simulink model "PVtestsiteeight"  (Simulink 10.1)
settings: Solver=FixedStepDiscrete  StartTime=0.0  StopTime=inf  FixedStep=Ts  RelTol=1e-3
PreLoadFcn:
  | init_DCDCDCAC_new
InitFcn:
  | init_DCDCDCAC_new
undefined symbols (not defined in the file or in its folder): D1, Delta, I, Left, Right, type, V
libraries: powerlib x174, powerlib_meascontrol x3, ssn_lib x2, artemis x1
(part 2 of 3)

== system PVtestsiteeight/SS_Grid/704 - 720 Config 723 ==
  Pi Section Line : powerlib/Elements/Pi Section Line  LConnTagsString=__new0  RConnTagsString=__new0  Frequency=60  Resistance=0.803807  Inductance=0.0011064  Capacitance=1.23355e-07  Length=D  PiSections=1  Measurements=None
      settings: AttributesFormatString=\n  SourceProductBaseCode=PS
  Pi Section Line1 : powerlib/Elements/Pi Section Line  LConnTagsString=__new0  RConnTagsString=__new0  Frequency=60  Resistance=0.80915157  Inductance=0.00104267  Capacitance=1.233552e-07  Length=D  PiSections=1  Measurements=None
      settings: AttributesFormatString=\n  SourceProductBaseCode=PS
  Pi Section Line2 : powerlib/Elements/Pi Section Line  LConnTagsString=__new0  RConnTagsString=__new0  Frequency=60  Resistance=0.8038077  Inductance=0.0011064  Capacitance=1.23355e-07  Length=D  PiSections=1  Measurements=None
      settings: AttributesFormatString=\n  SourceProductBaseCode=PS
  a : PMIOPort  Side=Left
  A : PMIOPort  Port=2  Side=Right
  b : PMIOPort  Port=3  Side=Left
  B : PMIOPort  Port=4  Side=Right
  c : PMIOPort  Port=5  Side=Left
  C : PMIOPort  Port=6  Side=Right
  connections:
  a/RConn1 -- Pi Section Line/LConn1
  A/RConn1 -- Pi Section Line/RConn1
  b/RConn1 -- Pi Section Line1/LConn1
  B/RConn1 -- Pi Section Line1/RConn1
  c/RConn1 -- Pi Section Line2/LConn1
  C/RConn1 -- Pi Section Line2/RConn1

== system PVtestsiteeight/SS_Grid/705 ==
  Three-Phase V-I Measurement : powerlib/Measurements/Three-Phase V-I Measurement  VoltageMeasurement=phase-to-ground  SetLabelV=off  LabelV=Vabc  Vpu=off  VpuLL=off  CurrentMeasurement=yes  SetLabelI=off  LabelI=Iabc  Ipu=off  Pbase=100e6  Vbase=500e3  OutputType=Complex  PhasorSimulation=off  PSBequivalent=0
  Conn1 : PMIOPort  Side=Left
  Conn2 : PMIOPort  Port=2  Side=Left
  Conn3 : PMIOPort  Port=3  Side=Right
  Conn4 : PMIOPort  Port=4  Side=Right
  Conn5 : PMIOPort  Port=5  Side=Left
  Conn6 : PMIOPort  Port=6  Side=Right
  tag scope: I_705=global, V_705=global
  wires:
  Three-Phase V-I Measurement/1 -> [V_705]
  Three-Phase V-I Measurement/2 -> [I_705]
  connections:
  Conn1/RConn1 -- Three-Phase V-I Measurement/LConn1
  Conn2/RConn1 -- Three-Phase V-I Measurement/LConn2
  Conn3/RConn1 -- Three-Phase V-I Measurement/RConn1
  Conn4/RConn1 -- Three-Phase V-I Measurement/RConn2
  Conn5/RConn1 -- Three-Phase V-I Measurement/LConn3
  Conn6/RConn1 -- Three-Phase V-I Measurement/RConn3

== system PVtestsiteeight/SS_Grid/705 - 712 config 724  ==
  Pi Section Line : powerlib/Elements/Pi Section Line  LConnTagsString=__new0  RConnTagsString=__new0  Frequency=60  Resistance=1.3019001  Inductance=0.0012787  Capacitance=9.93038e-08  Length=D  PiSections=1  Measurements=None
      settings: AttributesFormatString=\n  SourceProductBaseCode=PS
  Pi Section Line1 : powerlib/Elements/Pi Section Line  LConnTagsString=__new0  RConnTagsString=__new0  Frequency=60  Resistance=1.309108  Inductance=0.001219369  Capacitance=9.9303e-08  Length=D  PiSections=1  Measurements=None
      settings: AttributesFormatString=\n  SourceProductBaseCode=PS
  Pi Section Line2 : powerlib/Elements/Pi Section Line  LConnTagsString=__new0  RConnTagsString=__new0  Frequency=60  Resistance=1.3019001  Inductance=0.0012787  Capacitance=9.93038e-08  Length=D  PiSections=1  Measurements=None
      settings: AttributesFormatString=\n  SourceProductBaseCode=PS
  a : PMIOPort  Side=Left
  A : PMIOPort  Port=2  Side=Right
  b : PMIOPort  Port=3  Side=Left
  B : PMIOPort  Port=4  Side=Right
  c : PMIOPort  Port=5  Side=Left
  C : PMIOPort  Port=6  Side=Right
  connections:
  a/RConn1 -- Pi Section Line/LConn1
  A/RConn1 -- Pi Section Line/RConn1
  b/RConn1 -- Pi Section Line1/LConn1
  B/RConn1 -- Pi Section Line1/RConn1
  c/RConn1 -- Pi Section Line2/LConn1
  C/RConn1 -- Pi Section Line2/RConn1

== system PVtestsiteeight/SS_Grid/705 - 742 config 724 ==
  Pi Section Line : powerlib/Elements/Pi Section Line  LConnTagsString=__new0  RConnTagsString=__new0  Frequency=60  Resistance=1.3019001  Inductance=0.0012787  Capacitance=9.93038e-08  Length=D  PiSections=1  Measurements=None
      settings: AttributesFormatString=\n  SourceProductBaseCode=PS
  Pi Section Line1 : powerlib/Elements/Pi Section Line  LConnTagsString=__new0  RConnTagsString=__new0  Frequency=60  Resistance=1.309108  Inductance=0.001219369  Capacitance=9.9303e-08  Length=D  PiSections=1  Measurements=None
      settings: AttributesFormatString=\n  SourceProductBaseCode=PS
  Pi Section Line2 : powerlib/Elements/Pi Section Line  LConnTagsString=__new0  RConnTagsString=__new0  Frequency=60  Resistance=1.3019001  Inductance=0.0012787  Capacitance=9.93038e-08  Length=D  PiSections=1  Measurements=None
      settings: AttributesFormatString=\n  SourceProductBaseCode=PS
  a : PMIOPort  Side=Left
  A : PMIOPort  Port=2  Side=Right
  b : PMIOPort  Port=3  Side=Left
  B : PMIOPort  Port=4  Side=Right
  c : PMIOPort  Port=5  Side=Left
  C : PMIOPort  Port=6  Side=Right
  connections:
  C/RConn1 -- Pi Section Line2/RConn1
  c/RConn1 -- Pi Section Line2/LConn1
  B/RConn1 -- Pi Section Line1/RConn1
  b/RConn1 -- Pi Section Line1/LConn1
  A/RConn1 -- Pi Section Line/RConn1
  a/RConn1 -- Pi Section Line/LConn1

== system PVtestsiteeight/SS_Grid/706 ==
  Three-Phase V-I Measurement : powerlib/Measurements/Three-Phase V-I Measurement  VoltageMeasurement=phase-to-ground  SetLabelV=off  LabelV=Vabc  Vpu=off  VpuLL=off  CurrentMeasurement=yes  SetLabelI=off  LabelI=Iabc  Ipu=off  Pbase=100e6  Vbase=500e3  OutputType=Complex  PhasorSimulation=off  PSBequivalent=0
  Conn1 : PMIOPort  Side=Left
  Conn2 : PMIOPort  Port=2  Side=Left
  Conn3 : PMIOPort  Port=3  Side=Right
  Conn4 : PMIOPort  Port=4  Side=Right
  Conn5 : PMIOPort  Port=5  Side=Left
  Conn6 : PMIOPort  Port=6  Side=Right
  tag scope: I_706=global, V_706=global
  wires:
  Three-Phase V-I Measurement/2 -> [I_706]
  Three-Phase V-I Measurement/1 -> [V_706]
  connections:
  Conn6/RConn1 -- Three-Phase V-I Measurement/RConn3
  Conn5/RConn1 -- Three-Phase V-I Measurement/LConn3
  Conn4/RConn1 -- Three-Phase V-I Measurement/RConn2
  Conn3/RConn1 -- Three-Phase V-I Measurement/RConn1
  Conn2/RConn1 -- Three-Phase V-I Measurement/LConn2
  Conn1/RConn1 -- Three-Phase V-I Measurement/LConn1

== system PVtestsiteeight/SS_Grid/706 - 725  config 724 ==
  Pi Section Line : powerlib/Elements/Pi Section Line  LConnTagsString=__new0  RConnTagsString=__new0  Frequency=60  Resistance=1.3019001  Inductance=0.0012787  Capacitance=9.93038e-08  Length=D  PiSections=1  Measurements=None
      settings: AttributesFormatString=\n  SourceProductBaseCode=PS
  Pi Section Line1 : powerlib/Elements/Pi Section Line  LConnTagsString=__new0  RConnTagsString=__new0  Frequency=60  Resistance=1.309108  Inductance=0.001219369  Capacitance=9.9303e-08  Length=D  PiSections=1  Measurements=None
      settings: AttributesFormatString=\n  SourceProductBaseCode=PS
  Pi Section Line2 : powerlib/Elements/Pi Section Line  LConnTagsString=__new0  RConnTagsString=__new0  Frequency=60  Resistance=1.3019001  Inductance=0.0012787  Capacitance=9.93038e-08  Length=D  PiSections=1  Measurements=None
      settings: AttributesFormatString=\n  SourceProductBaseCode=PS
  a : PMIOPort  Side=Left
  A : PMIOPort  Port=2  Side=Right
  b : PMIOPort  Port=3  Side=Left
  B : PMIOPort  Port=4  Side=Right
  c : PMIOPort  Port=5  Side=Left
  C : PMIOPort  Port=6  Side=Right
  connections:
  C/RConn1 -- Pi Section Line2/RConn1
  c/RConn1 -- Pi Section Line2/LConn1
  B/RConn1 -- Pi Section Line1/RConn1
  b/RConn1 -- Pi Section Line1/LConn1
  A/RConn1 -- Pi Section Line/RConn1
  a/RConn1 -- Pi Section Line/LConn1

== system PVtestsiteeight/SS_Grid/707 ==
  Three-Phase V-I Measurement : powerlib/Measurements/Three-Phase V-I Measurement  VoltageMeasurement=phase-to-ground  SetLabelV=off  LabelV=Vabc  Vpu=off  VpuLL=off  CurrentMeasurement=yes  SetLabelI=off  LabelI=Iabc  Ipu=off  Pbase=100e6  Vbase=500e3  OutputType=Complex  PhasorSimulation=off  PSBequivalent=0
  Conn1 : PMIOPort  Side=Left
  Conn2 : PMIOPort  Port=2  Side=Left
  Conn3 : PMIOPort  Port=3  Side=Right
  Conn4 : PMIOPort  Port=4  Side=Right
  Conn5 : PMIOPort  Port=5  Side=Left
  Conn6 : PMIOPort  Port=6  Side=Right
  tag scope: I_707=global, V_707=global
  wires:
  Three-Phase V-I Measurement/1 -> [V_707]
  Three-Phase V-I Measurement/2 -> [I_707]
  connections:
  Conn1/RConn1 -- Three-Phase V-I Measurement/LConn1
  Conn2/RConn1 -- Three-Phase V-I Measurement/LConn2
  Conn3/RConn1 -- Three-Phase V-I Measurement/RConn1
  Conn4/RConn1 -- Three-Phase V-I Measurement/RConn2
  Conn5/RConn1 -- Three-Phase V-I Measurement/LConn3
  Conn6/RConn1 -- Three-Phase V-I Measurement/RConn3

== system PVtestsiteeight/SS_Grid/707 - 722 config 724 ==
  Pi Section Line : powerlib/Elements/Pi Section Line  LConnTagsString=__new0  RConnTagsString=__new0  Frequency=60  Resistance=1.3019001  Inductance=0.0012787  Capacitance=9.93038e-08  Length=D  PiSections=1  Measurements=None
      settings: AttributesFormatString=\n  SourceProductBaseCode=PS
  Pi Section Line1 : powerlib/Elements/Pi Section Line  LConnTagsString=__new0  RConnTagsString=__new0  Frequency=60  Resistance=1.309108  Inductance=0.001219369  Capacitance=9.9303e-08  Length=D  PiSections=1  Measurements=None
      settings: AttributesFormatString=\n  SourceProductBaseCode=PS
  Pi Section Line2 : powerlib/Elements/Pi Section Line  LConnTagsString=__new0  RConnTagsString=__new0  Frequency=60  Resistance=1.3019001  Inductance=0.0012787  Capacitance=9.93038e-08  Length=D  PiSections=1  Measurements=None
      settings: AttributesFormatString=\n  SourceProductBaseCode=PS
  a : PMIOPort  Side=Left
  A : PMIOPort  Port=2  Side=Right
  b : PMIOPort  Port=3  Side=Left
  B : PMIOPort  Port=4  Side=Right
  c : PMIOPort  Port=5  Side=Left
  C : PMIOPort  Port=6  Side=Right
  connections:
  a/RConn1 -- Pi Section Line/LConn1
  A/RConn1 -- Pi Section Line/RConn1
  b/RConn1 -- Pi Section Line1/LConn1
  B/RConn1 -- Pi Section Line1/RConn1
  c/RConn1 -- Pi Section Line2/LConn1
  C/RConn1 -- Pi Section Line2/RConn1

== system PVtestsiteeight/SS_Grid/707 - 724 config 724 ==
  Pi Section Line : powerlib/Elements/Pi Section Line  LConnTagsString=__new0  RConnTagsString=__new0  Frequency=60  Resistance=1.3019001  Inductance=0.0012787  Capacitance=9.93038e-08  Length=D  PiSections=1  Measurements=None
      settings: AttributesFormatString=\n  SourceProductBaseCode=PS
  Pi Section Line1 : powerlib/Elements/Pi Section Line  LConnTagsString=__new0  RConnTagsString=__new0  Frequency=60  Resistance=1.309108  Inductance=0.001219369  Capacitance=9.9303e-08  Length=D  PiSections=1  Measurements=None
      settings: AttributesFormatString=\n  SourceProductBaseCode=PS
  Pi Section Line2 : powerlib/Elements/Pi Section Line  LConnTagsString=__new0  RConnTagsString=__new0  Frequency=60  Resistance=1.3019001  Inductance=0.0012787  Capacitance=9.93038e-08  Length=D  PiSections=1  Measurements=None
      settings: AttributesFormatString=\n  SourceProductBaseCode=PS
  a : PMIOPort  Side=Left
  A : PMIOPort  Port=2  Side=Right
  b : PMIOPort  Port=3  Side=Left
  B : PMIOPort  Port=4  Side=Right
  c : PMIOPort  Port=5  Side=Left
  C : PMIOPort  Port=6  Side=Right
  connections:
  C/RConn1 -- Pi Section Line2/RConn1
  c/RConn1 -- Pi Section Line2/LConn1
  B/RConn1 -- Pi Section Line1/RConn1
  b/RConn1 -- Pi Section Line1/LConn1
  A/RConn1 -- Pi Section Line/RConn1
  a/RConn1 -- Pi Section Line/LConn1

== system PVtestsiteeight/SS_Grid/708 ==
  Three-Phase V-I Measurement : powerlib/Measurements/Three-Phase V-I Measurement  VoltageMeasurement=phase-to-ground  SetLabelV=off  LabelV=Vabc  Vpu=off  VpuLL=off  CurrentMeasurement=yes  SetLabelI=off  LabelI=Iabc  Ipu=off  Pbase=100e6  Vbase=500e3  OutputType=Complex  PhasorSimulation=off  PSBequivalent=0
  Conn1 : PMIOPort  Side=Left
  Conn2 : PMIOPort  Port=2  Side=Left
  Conn3 : PMIOPort  Port=3  Side=Right
  Conn4 : PMIOPort  Port=4  Side=Right
  Conn5 : PMIOPort  Port=5  Side=Left
  Conn6 : PMIOPort  Port=6  Side=Right
  tag scope: I_708=global, V_708=global
  wires:
  Three-Phase V-I Measurement/2 -> [I_708]
  Three-Phase V-I Measurement/1 -> [V_708]
  connections:
  Conn6/RConn1 -- Three-Phase V-I Measurement/RConn3
  Conn5/RConn1 -- Three-Phase V-I Measurement/LConn3
  Conn4/RConn1 -- Three-Phase V-I Measurement/RConn2
  Conn3/RConn1 -- Three-Phase V-I Measurement/RConn1
  Conn2/RConn1 -- Three-Phase V-I Measurement/LConn2
  Conn1/RConn1 -- Three-Phase V-I Measurement/LConn1

== system PVtestsiteeight/SS_Grid/708  - 733 Conf 723 ==
  Pi Section Line : powerlib/Elements/Pi Section Line  LConnTagsString=__new0  RConnTagsString=__new0  Frequency=60  Resistance=0.803807  Inductance=0.0011064  Capacitance=1.23355e-07  Length=D  PiSections=1  Measurements=None
      settings: AttributesFormatString=\n  SourceProductBaseCode=PS
  Pi Section Line1 : powerlib/Elements/Pi Section Line  LConnTagsString=__new0  RConnTagsString=__new0  Frequency=60  Resistance=0.80915157  Inductance=0.00104267  Capacitance=1.233552e-07  Length=D  PiSections=1  Measurements=None
      settings: AttributesFormatString=\n  SourceProductBaseCode=PS
  Pi Section Line2 : powerlib/Elements/Pi Section Line  LConnTagsString=__new0  RConnTagsString=__new0  Frequency=60  Resistance=0.8038077  Inductance=0.0011064  Capacitance=1.23355e-07  Length=D  PiSections=1  Measurements=None
      settings: AttributesFormatString=\n  SourceProductBaseCode=PS
  a : PMIOPort  Side=Left
  A : PMIOPort  Port=2  Side=Right
  b : PMIOPort  Port=3  Side=Left
  B : PMIOPort  Port=4  Side=Right
  c : PMIOPort  Port=5  Side=Left
  C : PMIOPort  Port=6  Side=Right
  connections:
  a/RConn1 -- Pi Section Line/LConn1
  A/RConn1 -- Pi Section Line/RConn1
  b/RConn1 -- Pi Section Line1/LConn1
  B/RConn1 -- Pi Section Line1/RConn1
  c/RConn1 -- Pi Section Line2/LConn1
  C/RConn1 -- Pi Section Line2/RConn1

== system PVtestsiteeight/SS_Grid/708- 732 config 724  ==
  Pi Section Line : powerlib/Elements/Pi Section Line  LConnTagsString=__new0  RConnTagsString=__new0  Frequency=60  Resistance=1.3019001  Inductance=0.0012787  Capacitance=9.93038e-08  Length=D  PiSections=1  Measurements=None
      settings: AttributesFormatString=\n  SourceProductBaseCode=PS
  Pi Section Line1 : powerlib/Elements/Pi Section Line  LConnTagsString=__new0  RConnTagsString=__new0  Frequency=60  Resistance=1.309108  Inductance=0.001219369  Capacitance=9.9303e-08  Length=D  PiSections=1  Measurements=None
      settings: AttributesFormatString=\n  SourceProductBaseCode=PS
  Pi Section Line2 : powerlib/Elements/Pi Section Line  LConnTagsString=__new0  RConnTagsString=__new0  Frequency=60  Resistance=1.3019001  Inductance=0.0012787  Capacitance=9.93038e-08  Length=D  PiSections=1  Measurements=None
      settings: AttributesFormatString=\n  SourceProductBaseCode=PS
  a : PMIOPort  Side=Left
  A : PMIOPort  Port=2  Side=Right
  b : PMIOPort  Port=3  Side=Left
  B : PMIOPort  Port=4  Side=Right
  c : PMIOPort  Port=5  Side=Left
  C : PMIOPort  Port=6  Side=Right
  connections:
  a/RConn1 -- Pi Section Line/LConn1
  A/RConn1 -- Pi Section Line/RConn1
  b/RConn1 -- Pi Section Line1/LConn1
  B/RConn1 -- Pi Section Line1/RConn1
  c/RConn1 -- Pi Section Line2/LConn1
  C/RConn1 -- Pi Section Line2/RConn1

== system PVtestsiteeight/SS_Grid/709 ==
  Three-Phase V-I Measurement : powerlib/Measurements/Three-Phase V-I Measurement  VoltageMeasurement=phase-to-ground  SetLabelV=off  LabelV=Vabc  Vpu=off  VpuLL=off  CurrentMeasurement=yes  SetLabelI=off  LabelI=Iabc  Ipu=off  Pbase=100e6  Vbase=500e3  OutputType=Complex  PhasorSimulation=off  PSBequivalent=0
  Conn1 : PMIOPort  Side=Left
  Conn2 : PMIOPort  Port=2  Side=Left
  Conn3 : PMIOPort  Port=3  Side=Right
  Conn4 : PMIOPort  Port=4  Side=Right
  Conn5 : PMIOPort  Port=5  Side=Left
  Conn6 : PMIOPort  Port=6  Side=Right
  tag scope: I_709=global, V_709=global
  wires:
  Three-Phase V-I Measurement/1 -> [V_709]
  Three-Phase V-I Measurement/2 -> [I_709]
  connections:
  Conn1/RConn1 -- Three-Phase V-I Measurement/LConn1
  Conn2/RConn1 -- Three-Phase V-I Measurement/LConn2
  Conn3/RConn1 -- Three-Phase V-I Measurement/RConn1
  Conn4/RConn1 -- Three-Phase V-I Measurement/RConn2
  Conn5/RConn1 -- Three-Phase V-I Measurement/LConn3
  Conn6/RConn1 -- Three-Phase V-I Measurement/RConn3

== system PVtestsiteeight/SS_Grid/709 - 708 Config 723 ==
  Pi Section Line : powerlib/Elements/Pi Section Line  LConnTagsString=__new0  RConnTagsString=__new0  Frequency=60  Resistance=0.803807  Inductance=0.0011064  Capacitance=1.23355e-07  Length=D  PiSections=1  Measurements=None
      settings: AttributesFormatString=\n  SourceProductBaseCode=PS
  Pi Section Line1 : powerlib/Elements/Pi Section Line  LConnTagsString=__new0  RConnTagsString=__new0  Frequency=60  Resistance=0.80915157  Inductance=0.00104267  Capacitance=1.233552e-07  Length=D  PiSections=1  Measurements=None
      settings: AttributesFormatString=\n  SourceProductBaseCode=PS
  Pi Section Line2 : powerlib/Elements/Pi Section Line  LConnTagsString=__new0  RConnTagsString=__new0  Frequency=60  Resistance=0.8038077  Inductance=0.0011064  Capacitance=1.23355e-07  Length=D  PiSections=1  Measurements=None
      settings: AttributesFormatString=\n  SourceProductBaseCode=PS
  a : PMIOPort  Side=Left
  A : PMIOPort  Port=2  Side=Right
  b : PMIOPort  Port=3  Side=Left
  B : PMIOPort  Port=4  Side=Right
  c : PMIOPort  Port=5  Side=Left
  C : PMIOPort  Port=6  Side=Right
  connections:
  C/RConn1 -- Pi Section Line2/RConn1
  c/RConn1 -- Pi Section Line2/LConn1
  B/RConn1 -- Pi Section Line1/RConn1
  b/RConn1 -- Pi Section Line1/LConn1
  A/RConn1 -- Pi Section Line/RConn1
  a/RConn1 -- Pi Section Line/LConn1

== system PVtestsiteeight/SS_Grid/709 - 731 Config 723 ==
  Pi Section Line : powerlib/Elements/Pi Section Line  LConnTagsString=__new0  RConnTagsString=__new0  Frequency=60  Resistance=0.803807  Inductance=0.0011064  Capacitance=1.23355e-07  Length=D  PiSections=1  Measurements=None
      settings: AttributesFormatString=\n  SourceProductBaseCode=PS
  Pi Section Line1 : powerlib/Elements/Pi Section Line  LConnTagsString=__new0  RConnTagsString=__new0  Frequency=60  Resistance=0.80915157  Inductance=0.00104267  Capacitance=1.233552e-07  Length=D  PiSections=1  Measurements=None
      settings: AttributesFormatString=\n  SourceProductBaseCode=PS
  Pi Section Line2 : powerlib/Elements/Pi Section Line  LConnTagsString=__new0  RConnTagsString=__new0  Frequency=60  Resistance=0.8038077  Inductance=0.0011064  Capacitance=1.23355e-07  Length=D  PiSections=1  Measurements=None
      settings: AttributesFormatString=\n  SourceProductBaseCode=PS
  a : PMIOPort  Side=Left
  A : PMIOPort  Port=2  Side=Right
  b : PMIOPort  Port=3  Side=Left
  B : PMIOPort  Port=4  Side=Right
  c : PMIOPort  Port=5  Side=Left
  C : PMIOPort  Port=6  Side=Right
  connections:
  a/RConn1 -- Pi Section Line/LConn1
  A/RConn1 -- Pi Section Line/RConn1
  b/RConn1 -- Pi Section Line1/LConn1
  B/RConn1 -- Pi Section Line1/RConn1
  c/RConn1 -- Pi Section Line2/LConn1
  C/RConn1 -- Pi Section Line2/RConn1

== system PVtestsiteeight/SS_Grid/710 ==
  Three-Phase V-I Measurement : powerlib/Measurements/Three-Phase V-I Measurement  VoltageMeasurement=phase-to-ground  SetLabelV=off  LabelV=Vabc  Vpu=off  VpuLL=off  CurrentMeasurement=yes  SetLabelI=off  LabelI=Iabc  Ipu=off  Pbase=100e6  Vbase=500e3  OutputType=Complex  PhasorSimulation=off  PSBequivalent=0
  Conn1 : PMIOPort  Side=Left
  Conn2 : PMIOPort  Port=2  Side=Left
  Conn3 : PMIOPort  Port=3  Side=Right
  Conn4 : PMIOPort  Port=4  Side=Right
  Conn5 : PMIOPort  Port=5  Side=Left
  Conn6 : PMIOPort  Port=6  Side=Right
  tag scope: I_710=global, V_710=global
  wires:
  Three-Phase V-I Measurement/2 -> [I_710]
  Three-Phase V-I Measurement/1 -> [V_710]
  connections:
  Conn6/RConn1 -- Three-Phase V-I Measurement/RConn3
  Conn5/RConn1 -- Three-Phase V-I Measurement/LConn3
  Conn4/RConn1 -- Three-Phase V-I Measurement/RConn2
  Conn3/RConn1 -- Three-Phase V-I Measurement/RConn1
  Conn2/RConn1 -- Three-Phase V-I Measurement/LConn2
  Conn1/RConn1 -- Three-Phase V-I Measurement/LConn1

== system PVtestsiteeight/SS_Grid/710 - 735 config 724  ==
  Pi Section Line : powerlib/Elements/Pi Section Line  LConnTagsString=__new0  RConnTagsString=__new0  Frequency=60  Resistance=1.3019001  Inductance=0.0012787  Capacitance=9.93038e-08  Length=D  PiSections=1  Measurements=None
      settings: AttributesFormatString=\n  SourceProductBaseCode=PS
  Pi Section Line1 : powerlib/Elements/Pi Section Line  LConnTagsString=__new0  RConnTagsString=__new0  Frequency=60  Resistance=1.309108  Inductance=0.001219369  Capacitance=9.9303e-08  Length=D  PiSections=1  Measurements=None
      settings: AttributesFormatString=\n  SourceProductBaseCode=PS
  Pi Section Line2 : powerlib/Elements/Pi Section Line  LConnTagsString=__new0  RConnTagsString=__new0  Frequency=60  Resistance=1.3019001  Inductance=0.0012787  Capacitance=9.93038e-08  Length=D  PiSections=1  Measurements=None
      settings: AttributesFormatString=\n  SourceProductBaseCode=PS
  a : PMIOPort  Side=Left
  A : PMIOPort  Port=2  Side=Right
  b : PMIOPort  Port=3  Side=Left
  B : PMIOPort  Port=4  Side=Right
  c : PMIOPort  Port=5  Side=Left
  C : PMIOPort  Port=6  Side=Right
  connections:
  C/RConn1 -- Pi Section Line2/RConn1
  c/RConn1 -- Pi Section Line2/LConn1
  B/RConn1 -- Pi Section Line1/RConn1
  b/RConn1 -- Pi Section Line1/LConn1
  A/RConn1 -- Pi Section Line/RConn1
  a/RConn1 -- Pi Section Line/LConn1

== system PVtestsiteeight/SS_Grid/710 - 736 config 724  ==
  Pi Section Line : powerlib/Elements/Pi Section Line  LConnTagsString=__new0  RConnTagsString=__new0  Frequency=60  Resistance=1.3019001  Inductance=0.0012787  Capacitance=9.93038e-08  Length=D  PiSections=1  Measurements=None
      settings: AttributesFormatString=\n  SourceProductBaseCode=PS
  Pi Section Line1 : powerlib/Elements/Pi Section Line  LConnTagsString=__new0  RConnTagsString=__new0  Frequency=60  Resistance=1.309108  Inductance=0.001219369  Capacitance=9.9303e-08  Length=D  PiSections=1  Measurements=None
      settings: AttributesFormatString=\n  SourceProductBaseCode=PS
  Pi Section Line2 : powerlib/Elements/Pi Section Line  LConnTagsString=__new0  RConnTagsString=__new0  Frequency=60  Resistance=1.3019001  Inductance=0.0012787  Capacitance=9.93038e-08  Length=D  PiSections=1  Measurements=None
      settings: AttributesFormatString=\n  SourceProductBaseCode=PS
  a : PMIOPort  Side=Left
  A : PMIOPort  Port=2  Side=Right
  b : PMIOPort  Port=3  Side=Left
  B : PMIOPort  Port=4  Side=Right
  c : PMIOPort  Port=5  Side=Left
  C : PMIOPort  Port=6  Side=Right
  connections:
  C/RConn1 -- Pi Section Line2/RConn1
  c/RConn1 -- Pi Section Line2/LConn1
  B/RConn1 -- Pi Section Line1/RConn1
  b/RConn1 -- Pi Section Line1/LConn1
  A/RConn1 -- Pi Section Line/RConn1
  a/RConn1 -- Pi Section Line/LConn1

== system PVtestsiteeight/SS_Grid/711 ==
  Three-Phase V-I Measurement : powerlib/Measurements/Three-Phase V-I Measurement  VoltageMeasurement=phase-to-ground  SetLabelV=off  LabelV=Vabc  Vpu=off  VpuLL=off  CurrentMeasurement=yes  SetLabelI=off  LabelI=Iabc  Ipu=off  Pbase=100e6  Vbase=500e3  OutputType=Complex  PhasorSimulation=off  PSBequivalent=0
  Conn1 : PMIOPort  Side=Left
  Conn2 : PMIOPort  Port=2  Side=Left
  Conn3 : PMIOPort  Port=3  Side=Right
  Conn4 : PMIOPort  Port=4  Side=Right
  Conn5 : PMIOPort  Port=5  Side=Left
  Conn6 : PMIOPort  Port=6  Side=Right
  tag scope: I_711=global, V_711=global
  wires:
  Three-Phase V-I Measurement/1 -> [V_711]
  Three-Phase V-I Measurement/2 -> [I_711]
  connections:
  Conn1/RConn1 -- Three-Phase V-I Measurement/LConn1
  Conn2/RConn1 -- Three-Phase V-I Measurement/LConn2
  Conn3/RConn1 -- Three-Phase V-I Measurement/RConn1
  Conn4/RConn1 -- Three-Phase V-I Measurement/RConn2
  Conn5/RConn1 -- Three-Phase V-I Measurement/LConn3
  Conn6/RConn1 -- Three-Phase V-I Measurement/RConn3

== system PVtestsiteeight/SS_Grid/711 - 740 config 724  ==
  Pi Section Line : powerlib/Elements/Pi Section Line  LConnTagsString=__new0  RConnTagsString=__new0  Frequency=60  Resistance=1.3019001  Inductance=0.0012787  Capacitance=9.93038e-08  Length=D  PiSections=1  Measurements=None
      settings: AttributesFormatString=\n  SourceProductBaseCode=PS
  Pi Section Line1 : powerlib/Elements/Pi Section Line  LConnTagsString=__new0  RConnTagsString=__new0  Frequency=60  Resistance=1.309108  Inductance=0.001219369  Capacitance=9.9303e-08  Length=D  PiSections=1  Measurements=None
      settings: AttributesFormatString=\n  SourceProductBaseCode=PS
  Pi Section Line2 : powerlib/Elements/Pi Section Line  LConnTagsString=__new0  RConnTagsString=__new0  Frequency=60  Resistance=1.3019001  Inductance=0.0012787  Capacitance=9.93038e-08  Length=D  PiSections=1  Measurements=None
      settings: AttributesFormatString=\n  SourceProductBaseCode=PS
  a : PMIOPort  Side=Left
  A : PMIOPort  Port=2  Side=Right
  b : PMIOPort  Port=3  Side=Left
  B : PMIOPort  Port=4  Side=Right
  c : PMIOPort  Port=5  Side=Left
  C : PMIOPort  Port=6  Side=Right
  connections:
  a/RConn1 -- Pi Section Line/LConn1
  A/RConn1 -- Pi Section Line/RConn1
  b/RConn1 -- Pi Section Line1/LConn1
  B/RConn1 -- Pi Section Line1/RConn1
  c/RConn1 -- Pi Section Line2/LConn1
  C/RConn1 -- Pi Section Line2/RConn1

== system PVtestsiteeight/SS_Grid/711 - 741 Conf 723  ==
  Pi Section Line : powerlib/Elements/Pi Section Line  LConnTagsString=__new0  RConnTagsString=__new0  Frequency=60  Resistance=0.803807  Inductance=0.0011064  Capacitance=1.23355e-07  Length=D  PiSections=1  Measurements=None
      settings: AttributesFormatString=\n  SourceProductBaseCode=PS
  Pi Section Line1 : powerlib/Elements/Pi Section Line  LConnTagsString=__new0  RConnTagsString=__new0  Frequency=60  Resistance=0.80915157  Inductance=0.00104267  Capacitance=1.233552e-07  Length=D  PiSections=1  Measurements=None
      settings: AttributesFormatString=\n  SourceProductBaseCode=PS
  Pi Section Line2 : powerlib/Elements/Pi Section Line  LConnTagsString=__new0  RConnTagsString=__new0  Frequency=60  Resistance=0.8038077  Inductance=0.0011064  Capacitance=1.23355e-07  Length=D  PiSections=1  Measurements=None
      settings: AttributesFormatString=\n  SourceProductBaseCode=PS
  a : PMIOPort  Side=Left
  A : PMIOPort  Port=2  Side=Right
  b : PMIOPort  Port=3  Side=Left
  B : PMIOPort  Port=4  Side=Right
  c : PMIOPort  Port=5  Side=Left
  C : PMIOPort  Port=6  Side=Right
  connections:
  C/RConn1 -- Pi Section Line2/RConn1
  c/RConn1 -- Pi Section Line2/LConn1
  B/RConn1 -- Pi Section Line1/RConn1
  b/RConn1 -- Pi Section Line1/LConn1
  A/RConn1 -- Pi Section Line/RConn1
  a/RConn1 -- Pi Section Line/LConn1

== system PVtestsiteeight/SS_Grid/712 ==
  Three-Phase V-I Measurement : powerlib/Measurements/Three-Phase V-I Measurement  VoltageMeasurement=phase-to-ground  SetLabelV=off  LabelV=Vabc  Vpu=off  VpuLL=off  CurrentMeasurement=yes  SetLabelI=off  LabelI=Iabc  Ipu=off  Pbase=100e6  Vbase=500e3  OutputType=Complex  PhasorSimulation=off  PSBequivalent=0
  Conn1 : PMIOPort  Side=Left
  Conn2 : PMIOPort  Port=2  Side=Left
  Conn3 : PMIOPort  Port=3  Side=Right
  Conn4 : PMIOPort  Port=4  Side=Right
  Conn5 : PMIOPort  Port=5  Side=Left
  Conn6 : PMIOPort  Port=6  Side=Right
  tag scope: I_712=global, V_712=global
  wires:
  Three-Phase V-I Measurement/1 -> [V_712]
  Three-Phase V-I Measurement/2 -> [I_712]
  connections:
  Conn1/RConn1 -- Three-Phase V-I Measurement/LConn1
  Conn2/RConn1 -- Three-Phase V-I Measurement/LConn2
  Conn3/RConn1 -- Three-Phase V-I Measurement/RConn1
  Conn4/RConn1 -- Three-Phase V-I Measurement/RConn2
  Conn5/RConn1 -- Three-Phase V-I Measurement/LConn3
  Conn6/RConn1 -- Three-Phase V-I Measurement/RConn3

== system PVtestsiteeight/SS_Grid/713 ==
  Three-Phase V-I Measurement : powerlib/Measurements/Three-Phase V-I Measurement  VoltageMeasurement=phase-to-ground  SetLabelV=off  LabelV=Vabc  Vpu=off  VpuLL=off  CurrentMeasurement=yes  SetLabelI=off  LabelI=Iabc  Ipu=off  Pbase=100e6  Vbase=500e3  OutputType=Complex  PhasorSimulation=off  PSBequivalent=0
  Conn1 : PMIOPort  Side=Left
  Conn2 : PMIOPort  Port=2  Side=Left
  Conn3 : PMIOPort  Port=3  Side=Right
  Conn4 : PMIOPort  Port=4  Side=Right
  Conn5 : PMIOPort  Port=5  Side=Left
  Conn6 : PMIOPort  Port=6  Side=Right
  tag scope: I_713=global, V_713=global
  wires:
  Three-Phase V-I Measurement/1 -> [V_713]
  Three-Phase V-I Measurement/2 -> [I_713]
  connections:
  Conn1/RConn1 -- Three-Phase V-I Measurement/LConn1
  Conn2/RConn1 -- Three-Phase V-I Measurement/LConn2
  Conn3/RConn1 -- Three-Phase V-I Measurement/RConn1
  Conn4/RConn1 -- Three-Phase V-I Measurement/RConn2
  Conn5/RConn1 -- Three-Phase V-I Measurement/LConn3
  Conn6/RConn1 -- Three-Phase V-I Measurement/RConn3

== system PVtestsiteeight/SS_Grid/713 - 704 Config 723 ==
  Pi Section Line : powerlib/Elements/Pi Section Line  LConnTagsString=__new0  RConnTagsString=__new0  Frequency=60  Resistance=0.803807  Inductance=0.0011064  Capacitance=1.23355e-07  Length=D  PiSections=1  Measurements=None
      settings: AttributesFormatString=\n  SourceProductBaseCode=PS
  Pi Section Line1 : powerlib/Elements/Pi Section Line  LConnTagsString=__new0  RConnTagsString=__new0  Frequency=60  Resistance=0.80915157  Inductance=0.00104267  Capacitance=1.233552e-07  Length=D  PiSections=1  Measurements=None
      settings: AttributesFormatString=\n  SourceProductBaseCode=PS
  Pi Section Line2 : powerlib/Elements/Pi Section Line  LConnTagsString=__new0  RConnTagsString=__new0  Frequency=60  Resistance=0.8038077  Inductance=0.0011064  Capacitance=1.23355e-07  Length=D  PiSections=1  Measurements=None
      settings: AttributesFormatString=\n  SourceProductBaseCode=PS
  a : PMIOPort  Side=Left
  A : PMIOPort  Port=2  Side=Right
  b : PMIOPort  Port=3  Side=Left
  B : PMIOPort  Port=4  Side=Right
  c : PMIOPort  Port=5  Side=Left
  C : PMIOPort  Port=6  Side=Right
  connections:
  C/RConn1 -- Pi Section Line2/RConn1
  c/RConn1 -- Pi Section Line2/LConn1
  B/RConn1 -- Pi Section Line1/RConn1
  b/RConn1 -- Pi Section Line1/LConn1
  A/RConn1 -- Pi Section Line/RConn1
  a/RConn1 -- Pi Section Line/LConn1

== system PVtestsiteeight/SS_Grid/714 ==
  Three-Phase V-I Measurement : powerlib/Measurements/Three-Phase V-I Measurement  VoltageMeasurement=phase-to-ground  SetLabelV=off  LabelV=Vabc  Vpu=off  VpuLL=off  CurrentMeasurement=yes  SetLabelI=off  LabelI=Iabc  Ipu=off  Pbase=100e6  Vbase=500e3  OutputType=Complex  PhasorSimulation=off  PSBequivalent=0
  Conn1 : PMIOPort  Side=Left
  Conn2 : PMIOPort  Port=2  Side=Left
  Conn3 : PMIOPort  Port=3  Side=Right
  Conn4 : PMIOPort  Port=4  Side=Right
  Conn5 : PMIOPort  Port=5  Side=Left
  Conn6 : PMIOPort  Port=6  Side=Right
  tag scope: I_714=global, V_714=global
  wires:
  Three-Phase V-I Measurement/1 -> [V_714]
  Three-Phase V-I Measurement/2 -> [I_714]
  connections:
  Conn1/RConn1 -- Three-Phase V-I Measurement/LConn1
  Conn2/RConn1 -- Three-Phase V-I Measurement/LConn2
  Conn3/RConn1 -- Three-Phase V-I Measurement/RConn1
  Conn4/RConn1 -- Three-Phase V-I Measurement/RConn2
  Conn5/RConn1 -- Three-Phase V-I Measurement/LConn3
  Conn6/RConn1 -- Three-Phase V-I Measurement/RConn3

== system PVtestsiteeight/SS_Grid/714 - 718  config 724 ==
  Pi Section Line : powerlib/Elements/Pi Section Line  LConnTagsString=__new0  RConnTagsString=__new0  Frequency=60  Resistance=1.3019001  Inductance=0.0012787  Capacitance=9.93038e-08  Length=D  PiSections=1  Measurements=None
      settings: AttributesFormatString=\n  SourceProductBaseCode=PS
  Pi Section Line1 : powerlib/Elements/Pi Section Line  LConnTagsString=__new0  RConnTagsString=__new0  Frequency=60  Resistance=1.309108  Inductance=0.001219369  Capacitance=9.9303e-08  Length=D  PiSections=1  Measurements=None
      settings: AttributesFormatString=\n  SourceProductBaseCode=PS
  Pi Section Line2 : powerlib/Elements/Pi Section Line  LConnTagsString=__new0  RConnTagsString=__new0  Frequency=60  Resistance=1.3019001  Inductance=0.0012787  Capacitance=9.93038e-08  Length=D  PiSections=1  Measurements=None
      settings: AttributesFormatString=\n  SourceProductBaseCode=PS
  a : PMIOPort  Side=Left
  A : PMIOPort  Port=2  Side=Right
  b : PMIOPort  Port=3  Side=Left
  B : PMIOPort  Port=4  Side=Right
  c : PMIOPort  Port=5  Side=Left
  C : PMIOPort  Port=6  Side=Right
  connections:
  a/RConn1 -- Pi Section Line/LConn1
  A/RConn1 -- Pi Section Line/RConn1
  b/RConn1 -- Pi Section Line1/LConn1
  B/RConn1 -- Pi Section Line1/RConn1
  c/RConn1 -- Pi Section Line2/LConn1
  C/RConn1 -- Pi Section Line2/RConn1

== system PVtestsiteeight/SS_Grid/718 ==
  Three-Phase V-I Measurement : powerlib/Measurements/Three-Phase V-I Measurement  VoltageMeasurement=phase-to-ground  SetLabelV=off  LabelV=Vabc  Vpu=off  VpuLL=off  CurrentMeasurement=yes  SetLabelI=off  LabelI=Iabc  Ipu=off  Pbase=100e6  Vbase=500e3  OutputType=Complex  PhasorSimulation=off  PSBequivalent=0
  Conn1 : PMIOPort  Side=Left
  Conn2 : PMIOPort  Port=2  Side=Left
  Conn3 : PMIOPort  Port=3  Side=Right
  Conn4 : PMIOPort  Port=4  Side=Right
  Conn5 : PMIOPort  Port=5  Side=Left
  Conn6 : PMIOPort  Port=6  Side=Right
  tag scope: I_718=global, V_718=global
  wires:
  Three-Phase V-I Measurement/2 -> [I_718]
  Three-Phase V-I Measurement/1 -> [V_718]
  connections:
  Conn6/RConn1 -- Three-Phase V-I Measurement/RConn3
  Conn5/RConn1 -- Three-Phase V-I Measurement/LConn3
  Conn4/RConn1 -- Three-Phase V-I Measurement/RConn2
  Conn3/RConn1 -- Three-Phase V-I Measurement/RConn1
  Conn2/RConn1 -- Three-Phase V-I Measurement/LConn2
  Conn1/RConn1 -- Three-Phase V-I Measurement/LConn1

== system PVtestsiteeight/SS_Grid/720 ==
  Three-Phase V-I Measurement : powerlib/Measurements/Three-Phase V-I Measurement  VoltageMeasurement=phase-to-ground  SetLabelV=off  LabelV=Vabc  Vpu=off  VpuLL=off  CurrentMeasurement=yes  SetLabelI=off  LabelI=Iabc  Ipu=off  Pbase=100e6  Vbase=500e3  OutputType=Complex  PhasorSimulation=off  PSBequivalent=0
  Conn1 : PMIOPort  Side=Left
  Conn2 : PMIOPort  Port=2  Side=Left
  Conn3 : PMIOPort  Port=3  Side=Right
  Conn4 : PMIOPort  Port=4  Side=Right
  Conn5 : PMIOPort  Port=5  Side=Left
  Conn6 : PMIOPort  Port=6  Side=Right
  tag scope: I_720=global, V_720=global
  wires:
  Three-Phase V-I Measurement/1 -> [V_720]
  Three-Phase V-I Measurement/2 -> [I_720]
  connections:
  Conn1/RConn1 -- Three-Phase V-I Measurement/LConn1
  Conn2/RConn1 -- Three-Phase V-I Measurement/LConn2
  Conn3/RConn1 -- Three-Phase V-I Measurement/RConn1
  Conn4/RConn1 -- Three-Phase V-I Measurement/RConn2
  Conn5/RConn1 -- Three-Phase V-I Measurement/LConn3
  Conn6/RConn1 -- Three-Phase V-I Measurement/RConn3

== system PVtestsiteeight/SS_Grid/720  - 706 Config 723 ==
  Pi Section Line : powerlib/Elements/Pi Section Line  LConnTagsString=__new0  RConnTagsString=__new0  Frequency=60  Resistance=0.803807  Inductance=0.0011064  Capacitance=1.23355e-07  Length=D  PiSections=1  Measurements=None
      settings: AttributesFormatString=\n  SourceProductBaseCode=PS
  Pi Section Line1 : powerlib/Elements/Pi Section Line  LConnTagsString=__new0  RConnTagsString=__new0  Frequency=60  Resistance=0.80915157  Inductance=0.00104267  Capacitance=1.233552e-07  Length=D  PiSections=1  Measurements=None
      settings: AttributesFormatString=\n  SourceProductBaseCode=PS
  Pi Section Line2 : powerlib/Elements/Pi Section Line  LConnTagsString=__new0  RConnTagsString=__new0  Frequency=60  Resistance=0.8038077  Inductance=0.0011064  Capacitance=1.23355e-07  Length=D  PiSections=1  Measurements=None
      settings: AttributesFormatString=\n  SourceProductBaseCode=PS
  a : PMIOPort  Side=Left
  A : PMIOPort  Port=2  Side=Right
  b : PMIOPort  Port=3  Side=Left
  B : PMIOPort  Port=4  Side=Right
  c : PMIOPort  Port=5  Side=Left
  C : PMIOPort  Port=6  Side=Right
  connections:
  C/RConn1 -- Pi Section Line2/RConn1
  c/RConn1 -- Pi Section Line2/LConn1
  B/RConn1 -- Pi Section Line1/RConn1
  b/RConn1 -- Pi Section Line1/LConn1
  A/RConn1 -- Pi Section Line/RConn1
  a/RConn1 -- Pi Section Line/LConn1

== system PVtestsiteeight/SS_Grid/720 - 707  config 724 ==
  Pi Section Line : powerlib/Elements/Pi Section Line  LConnTagsString=__new0  RConnTagsString=__new0  Frequency=60  Resistance=1.3019001  Inductance=0.0012787  Capacitance=9.93038e-08  Length=D  PiSections=1  Measurements=None
      settings: AttributesFormatString=\n  SourceProductBaseCode=PS
  Pi Section Line1 : powerlib/Elements/Pi Section Line  LConnTagsString=__new0  RConnTagsString=__new0  Frequency=60  Resistance=1.309108  Inductance=0.001219369  Capacitance=9.9303e-08  Length=D  PiSections=1  Measurements=None
      settings: AttributesFormatString=\n  SourceProductBaseCode=PS
  Pi Section Line2 : powerlib/Elements/Pi Section Line  LConnTagsString=__new0  RConnTagsString=__new0  Frequency=60  Resistance=1.3019001  Inductance=0.0012787  Capacitance=9.93038e-08  Length=D  PiSections=1  Measurements=None
      settings: AttributesFormatString=\n  SourceProductBaseCode=PS
  a : PMIOPort  Side=Left
  A : PMIOPort  Port=2  Side=Right
  b : PMIOPort  Port=3  Side=Left
  B : PMIOPort  Port=4  Side=Right
  c : PMIOPort  Port=5  Side=Left
  C : PMIOPort  Port=6  Side=Right
  connections:
  a/RConn1 -- Pi Section Line/LConn1
  A/RConn1 -- Pi Section Line/RConn1
  b/RConn1 -- Pi Section Line1/LConn1
  B/RConn1 -- Pi Section Line1/RConn1
  c/RConn1 -- Pi Section Line2/LConn1
  C/RConn1 -- Pi Section Line2/RConn1

== system PVtestsiteeight/SS_Grid/722 ==
  Three-Phase V-I Measurement : powerlib/Measurements/Three-Phase V-I Measurement  VoltageMeasurement=phase-to-ground  SetLabelV=off  LabelV=Vabc  Vpu=off  VpuLL=off  CurrentMeasurement=yes  SetLabelI=off  LabelI=Iabc  Ipu=off  Pbase=100e6  Vbase=500e3  OutputType=Complex  PhasorSimulation=off  PSBequivalent=0
  Conn1 : PMIOPort  Side=Left
  Conn2 : PMIOPort  Port=2  Side=Left
  Conn3 : PMIOPort  Port=3  Side=Right
  Conn4 : PMIOPort  Port=4  Side=Right
  Conn5 : PMIOPort  Port=5  Side=Left
  Conn6 : PMIOPort  Port=6  Side=Right
  tag scope: I_722=global, V_722=global
  wires:
  Three-Phase V-I Measurement/2 -> [I_722]
  Three-Phase V-I Measurement/1 -> [V_722]
  connections:
  Conn6/RConn1 -- Three-Phase V-I Measurement/RConn3
  Conn5/RConn1 -- Three-Phase V-I Measurement/LConn3
  Conn4/RConn1 -- Three-Phase V-I Measurement/RConn2
  Conn3/RConn1 -- Three-Phase V-I Measurement/RConn1
  Conn2/RConn1 -- Three-Phase V-I Measurement/LConn2
  Conn1/RConn1 -- Three-Phase V-I Measurement/LConn1

== system PVtestsiteeight/SS_Grid/724 ==
  Three-Phase V-I Measurement : powerlib/Measurements/Three-Phase V-I Measurement  VoltageMeasurement=phase-to-ground  SetLabelV=off  LabelV=Vabc  Vpu=off  VpuLL=off  CurrentMeasurement=yes  SetLabelI=off  LabelI=Iabc  Ipu=off  Pbase=100e6  Vbase=500e3  OutputType=Complex  PhasorSimulation=off  PSBequivalent=0
  Conn1 : PMIOPort  Side=Left
  Conn2 : PMIOPort  Port=2  Side=Left
  Conn3 : PMIOPort  Port=3  Side=Right
  Conn4 : PMIOPort  Port=4  Side=Right
  Conn5 : PMIOPort  Port=5  Side=Left
  Conn6 : PMIOPort  Port=6  Side=Right
  tag scope: I_724=global, V_724=global
  wires:
  Three-Phase V-I Measurement/2 -> [I_724]
  Three-Phase V-I Measurement/1 -> [V_724]
  connections:
  Conn6/RConn1 -- Three-Phase V-I Measurement/RConn3
  Conn5/RConn1 -- Three-Phase V-I Measurement/LConn3
  Conn4/RConn1 -- Three-Phase V-I Measurement/RConn2
  Conn3/RConn1 -- Three-Phase V-I Measurement/RConn1
  Conn2/RConn1 -- Three-Phase V-I Measurement/LConn2
  Conn1/RConn1 -- Three-Phase V-I Measurement/LConn1

== system PVtestsiteeight/SS_Grid/725 ==
  Three-Phase V-I Measurement : powerlib/Measurements/Three-Phase V-I Measurement  VoltageMeasurement=phase-to-ground  SetLabelV=off  LabelV=Vabc  Vpu=off  VpuLL=off  CurrentMeasurement=yes  SetLabelI=off  LabelI=Iabc  Ipu=off  Pbase=100e6  Vbase=500e3  OutputType=Complex  PhasorSimulation=off  PSBequivalent=0
  Conn1 : PMIOPort  Side=Left
  Conn2 : PMIOPort  Port=2  Side=Left
  Conn3 : PMIOPort  Port=3  Side=Right
  Conn4 : PMIOPort  Port=4  Side=Right
  Conn5 : PMIOPort  Port=5  Side=Left
  Conn6 : PMIOPort  Port=6  Side=Right
  tag scope: I_725=global, V_725=global
  wires:
  Three-Phase V-I Measurement/1 -> [V_725]
  Three-Phase V-I Measurement/2 -> [I_725]
  connections:
  Conn1/RConn1 -- Three-Phase V-I Measurement/LConn1
  Conn2/RConn1 -- Three-Phase V-I Measurement/LConn2
  Conn3/RConn1 -- Three-Phase V-I Measurement/RConn1
  Conn4/RConn1 -- Three-Phase V-I Measurement/RConn2
  Conn5/RConn1 -- Three-Phase V-I Measurement/LConn3
  Conn6/RConn1 -- Three-Phase V-I Measurement/RConn3

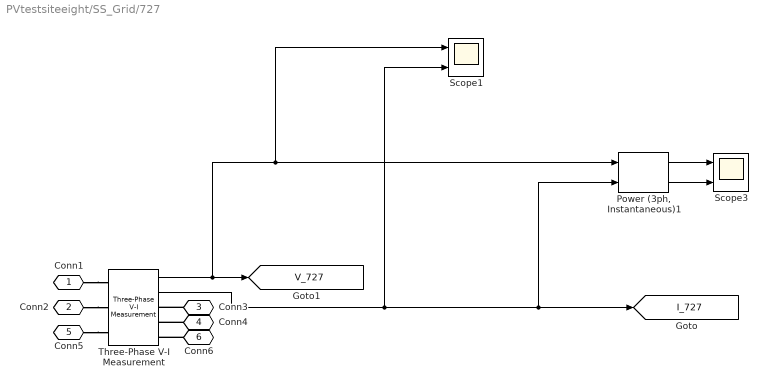
== system PVtestsiteeight/SS_Grid/727 ==
  "Power (3ph, Instantaneous)1" : powerlib_meascontrol/Measurements/Power (3ph, Instantaneous)
  Scope1 : Scope  NumInputPorts=2
  Scope3 : Scope  NumInputPorts=2
  Three-Phase V-I Measurement : powerlib/Measurements/Three-Phase V-I Measurement  VoltageMeasurement=phase-to-ground  SetLabelV=off  LabelV=Vabc  Vpu=off  VpuLL=off  CurrentMeasurement=yes  SetLabelI=off  LabelI=Iabc  Ipu=off  Pbase=100e6  Vbase=500e3  OutputType=Complex  PhasorSimulation=off  PSBequivalent=0
  Conn1 : PMIOPort  Side=Left
  Conn2 : PMIOPort  Port=2  Side=Left
  Conn3 : PMIOPort  Port=3  Side=Right
  Conn4 : PMIOPort  Port=4  Side=Right
  Conn5 : PMIOPort  Port=5  Side=Left
  Conn6 : PMIOPort  Port=6  Side=Right
  tag scope: I_727=global, V_727=global
  wires:
  "Power (3ph, Instantaneous)1"/1 -> Scope3/1
  "Power (3ph, Instantaneous)1"/2 -> Scope3/2
  Three-Phase V-I Measurement/1 -> Scope1/1, "Power (3ph, Instantaneous)1"/1, [V_727]
  Three-Phase V-I Measurement/2 -> Scope1/2, "Power (3ph, Instantaneous)1"/2, [I_727]
  connections:
  Conn1/RConn1 -- Three-Phase V-I Measurement/LConn1
  Conn2/RConn1 -- Three-Phase V-I Measurement/LConn2
  Conn3/RConn1 -- Three-Phase V-I Measurement/RConn1
  Conn4/RConn1 -- Three-Phase V-I Measurement/RConn2
  Conn5/RConn1 -- Three-Phase V-I Measurement/LConn3
  Conn6/RConn1 -- Three-Phase V-I Measurement/RConn3

== system PVtestsiteeight/SS_Grid/727 - 744 Config 723 ==
  Pi Section Line : powerlib/Elements/Pi Section Line  LConnTagsString=__new0  RConnTagsString=__new0  Frequency=60  Resistance=0.803807  Inductance=0.0011064  Capacitance=1.23355e-07  Length=D  PiSections=1  Measurements=None
      settings: AttributesFormatString=\n  SourceProductBaseCode=PS
  Pi Section Line1 : powerlib/Elements/Pi Section Line  LConnTagsString=__new0  RConnTagsString=__new0  Frequency=60  Resistance=0.80915157  Inductance=0.00104267  Capacitance=1.233552e-07  Length=D  PiSections=1  Measurements=None
      settings: AttributesFormatString=\n  SourceProductBaseCode=PS
  Pi Section Line2 : powerlib/Elements/Pi Section Line  LConnTagsString=__new0  RConnTagsString=__new0  Frequency=60  Resistance=0.8038077  Inductance=0.0011064  Capacitance=1.23355e-07  Length=D  PiSections=1  Measurements=None
      settings: AttributesFormatString=\n  SourceProductBaseCode=PS
  a : PMIOPort  Side=Left
  A : PMIOPort  Port=2  Side=Right
  b : PMIOPort  Port=3  Side=Left
  B : PMIOPort  Port=4  Side=Right
  c : PMIOPort  Port=5  Side=Left
  C : PMIOPort  Port=6  Side=Right
  connections:
  C/RConn1 -- Pi Section Line2/RConn1
  c/RConn1 -- Pi Section Line2/LConn1
  B/RConn1 -- Pi Section Line1/RConn1
  b/RConn1 -- Pi Section Line1/LConn1
  A/RConn1 -- Pi Section Line/RConn1
  a/RConn1 -- Pi Section Line/LConn1

== system PVtestsiteeight/SS_Grid/728 ==
  Three-Phase V-I Measurement : powerlib/Measurements/Three-Phase V-I Measurement  VoltageMeasurement=phase-to-ground  SetLabelV=off  LabelV=Vabc  Vpu=off  VpuLL=off  CurrentMeasurement=yes  SetLabelI=off  LabelI=Iabc  Ipu=off  Pbase=100e6  Vbase=500e3  OutputType=Complex  PhasorSimulation=off  PSBequivalent=0
  Conn1 : PMIOPort  Side=Left
  Conn2 : PMIOPort  Port=2  Side=Left
  Conn3 : PMIOPort  Port=3  Side=Right
  Conn4 : PMIOPort  Port=4  Side=Right
  Conn5 : PMIOPort  Port=5  Side=Left
  Conn6 : PMIOPort  Port=6  Side=Right
  tag scope: I_728=global, V_728=global
  wires:
  Three-Phase V-I Measurement/1 -> [V_728]
  Three-Phase V-I Measurement/2 -> [I_728]
  connections:
  Conn1/RConn1 -- Three-Phase V-I Measurement/LConn1
  Conn2/RConn1 -- Three-Phase V-I Measurement/LConn2
  Conn3/RConn1 -- Three-Phase V-I Measurement/RConn1
  Conn4/RConn1 -- Three-Phase V-I Measurement/RConn2
  Conn5/RConn1 -- Three-Phase V-I Measurement/LConn3
  Conn6/RConn1 -- Three-Phase V-I Measurement/RConn3

== system PVtestsiteeight/SS_Grid/730 ==
  Three-Phase V-I Measurement : powerlib/Measurements/Three-Phase V-I Measurement  VoltageMeasurement=phase-to-ground  SetLabelV=off  LabelV=Vabc  Vpu=off  VpuLL=off  CurrentMeasurement=yes  SetLabelI=off  LabelI=Iabc  Ipu=off  Pbase=100e6  Vbase=500e3  OutputType=Complex  PhasorSimulation=off  PSBequivalent=0
  Conn1 : PMIOPort  Side=Left
  Conn2 : PMIOPort  Port=2  Side=Left
  Conn3 : PMIOPort  Port=3  Side=Right
  Conn4 : PMIOPort  Port=4  Side=Right
  Conn5 : PMIOPort  Port=5  Side=Left
  Conn6 : PMIOPort  Port=6  Side=Right
  tag scope: I_730=global, V_730=global
  wires:
  Three-Phase V-I Measurement/2 -> [I_730]
  Three-Phase V-I Measurement/1 -> [V_730]
  connections:
  Conn6/RConn1 -- Three-Phase V-I Measurement/RConn3
  Conn5/RConn1 -- Three-Phase V-I Measurement/LConn3
  Conn4/RConn1 -- Three-Phase V-I Measurement/RConn2
  Conn3/RConn1 -- Three-Phase V-I Measurement/RConn1
  Conn2/RConn1 -- Three-Phase V-I Measurement/LConn2
  Conn1/RConn1 -- Three-Phase V-I Measurement/LConn1

== system PVtestsiteeight/SS_Grid/730 - 709 Config 723 ==
  Pi Section Line : powerlib/Elements/Pi Section Line  LConnTagsString=__new0  RConnTagsString=__new0  Frequency=60  Resistance=0.803807  Inductance=0.0011064  Capacitance=1.23355e-07  Length=D  PiSections=1  Measurements=None
      settings: AttributesFormatString=\n  SourceProductBaseCode=PS
  Pi Section Line1 : powerlib/Elements/Pi Section Line  LConnTagsString=__new0  RConnTagsString=__new0  Frequency=60  Resistance=0.80915157  Inductance=0.00104267  Capacitance=1.233552e-07  Length=D  PiSections=1  Measurements=None
      settings: AttributesFormatString=\n  SourceProductBaseCode=PS
  Pi Section Line2 : powerlib/Elements/Pi Section Line  LConnTagsString=__new0  RConnTagsString=__new0  Frequency=60  Resistance=0.8038077  Inductance=0.0011064  Capacitance=1.23355e-07  Length=D  PiSections=1  Measurements=None
      settings: AttributesFormatString=\n  SourceProductBaseCode=PS
  a : PMIOPort  Side=Left
  A : PMIOPort  Port=2  Side=Right
  b : PMIOPort  Port=3  Side=Left
  B : PMIOPort  Port=4  Side=Right
  c : PMIOPort  Port=5  Side=Left
  C : PMIOPort  Port=6  Side=Right
  connections:
  a/RConn1 -- Pi Section Line/LConn1
  A/RConn1 -- Pi Section Line/RConn1
  b/RConn1 -- Pi Section Line1/LConn1
  B/RConn1 -- Pi Section Line1/RConn1
  c/RConn1 -- Pi Section Line2/LConn1
  C/RConn1 -- Pi Section Line2/RConn1

== system PVtestsiteeight/SS_Grid/731 ==
  Three-Phase V-I Measurement : powerlib/Measurements/Three-Phase V-I Measurement  VoltageMeasurement=phase-to-ground  SetLabelV=off  LabelV=Vabc  Vpu=off  VpuLL=off  CurrentMeasurement=yes  SetLabelI=off  LabelI=Iabc  Ipu=off  Pbase=100e6  Vbase=500e3  OutputType=Complex  PhasorSimulation=off  PSBequivalent=0
  Conn1 : PMIOPort  Side=Left
  Conn2 : PMIOPort  Port=2  Side=Left
  Conn3 : PMIOPort  Port=3  Side=Right
  Conn4 : PMIOPort  Port=4  Side=Right
  Conn5 : PMIOPort  Port=5  Side=Left
  Conn6 : PMIOPort  Port=6  Side=Right
  tag scope: I_731=global, V_731=global
  wires:
  Three-Phase V-I Measurement/2 -> [I_731]
  Three-Phase V-I Measurement/1 -> [V_731]
  connections:
  Conn6/RConn1 -- Three-Phase V-I Measurement/RConn3
  Conn5/RConn1 -- Three-Phase V-I Measurement/LConn3
  Conn4/RConn1 -- Three-Phase V-I Measurement/RConn2
  Conn3/RConn1 -- Three-Phase V-I Measurement/RConn1
  Conn2/RConn1 -- Three-Phase V-I Measurement/LConn2
  Conn1/RConn1 -- Three-Phase V-I Measurement/LConn1

== system PVtestsiteeight/SS_Grid/732 ==
  Three-Phase V-I Measurement : powerlib/Measurements/Three-Phase V-I Measurement  VoltageMeasurement=phase-to-ground  SetLabelV=off  LabelV=Vabc  Vpu=off  VpuLL=off  CurrentMeasurement=yes  SetLabelI=off  LabelI=Iabc  Ipu=off  Pbase=100e6  Vbase=500e3  OutputType=Complex  PhasorSimulation=off  PSBequivalent=0
  Conn1 : PMIOPort  Side=Left
  Conn2 : PMIOPort  Port=2  Side=Left
  Conn3 : PMIOPort  Port=3  Side=Right
  Conn4 : PMIOPort  Port=4  Side=Right
  Conn5 : PMIOPort  Port=5  Side=Left
  Conn6 : PMIOPort  Port=6  Side=Right
  tag scope: I_732=global, V_732=global
  wires:
  Three-Phase V-I Measurement/1 -> [V_732]
  Three-Phase V-I Measurement/2 -> [I_732]
  connections:
  Conn1/RConn1 -- Three-Phase V-I Measurement/LConn1
  Conn2/RConn1 -- Three-Phase V-I Measurement/LConn2
  Conn3/RConn1 -- Three-Phase V-I Measurement/RConn1
  Conn4/RConn1 -- Three-Phase V-I Measurement/RConn2
  Conn5/RConn1 -- Three-Phase V-I Measurement/LConn3
  Conn6/RConn1 -- Three-Phase V-I Measurement/RConn3
